simulink model "VisualizationData"  (R2020a)
settings: Solver=VariableStepAuto  StartTime=0.0  StopTime=60  RelTol=1e-3
settings Model: Creator=kashy  LastModifiedBy=kashy

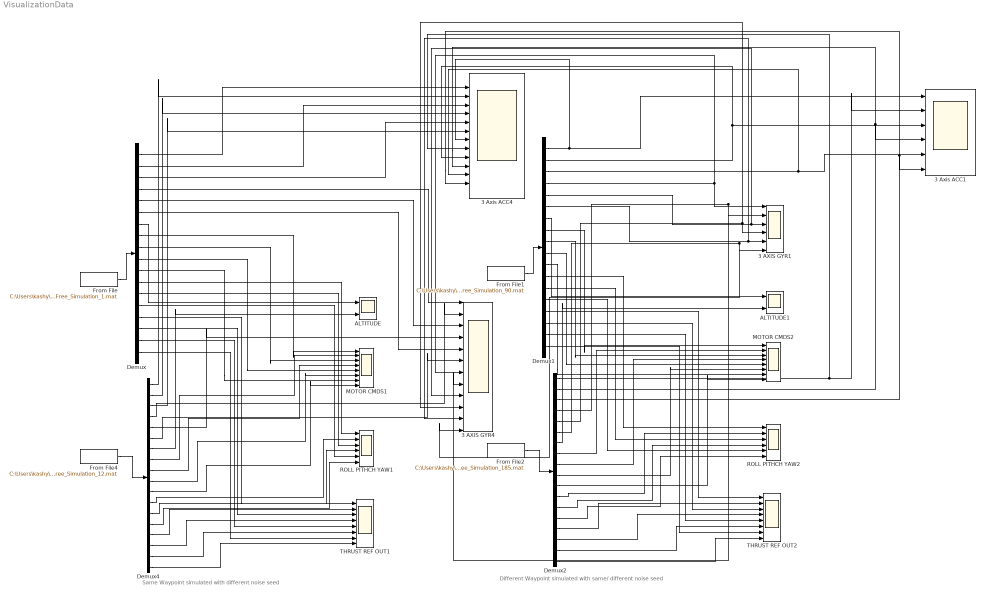
== system VisualizationData ==
  note: Same Waypoint simulated with different noise seed
  note: Different Waypoint simulated with same/ different noise seed
  3 AXIS GYR1 : Scope  NumInputPorts=6
  3 AXIS GYR4 : Scope  NumInputPorts=12
  3 Axis ACC1 : Scope  NumInputPorts=6
  3 Axis ACC4 : Scope  NumInputPorts=12
  ALTITUDE : Scope  NumInputPorts=2
  ALTITUDE1 : Scope  NumInputPorts=2
  Demux{,1..2,4} (4 alike) : Demux  Outputs=18
  From File : FromFile  FileName=C:\Users\kashy\Documents\MATLAB\Master_Thesis\model\parrotMinidroneWaypointFollower\Fault_Free_Data\Fault_Free_Simulation_1.mat  SampleTime=0.1
  From File1 : FromFile  FileName=C:\Users\kashy\Documents\MATLAB\Master_Thesis\model\parrotMinidroneWaypointFollower\Fault_Free_Data\Fault_Free_Simulation_90.mat  SampleTime=0.1
  From File2 : FromFile  FileName=C:\Users\kashy\Documents\MATLAB\Master_Thesis\model\parrotMinidroneWaypointFollower\Fault_Free_Data\Fault_Free_Simulation_185.mat  SampleTime=0.1
  From File4 : FromFile  FileName=C:\Users\kashy\Documents\MATLAB\Master_Thesis\model\parrotMinidroneWaypointFollower\Fault_Free_Data\Fault_Free_Simulation_12.mat  SampleTime=0.1
  MOTOR CMDS1 : Scope  NumInputPorts=8
  MOTOR CMDS2 : Scope  NumInputPorts=8
  ROLL PITHCH YAW1 : Scope  NumInputPorts=6
  ROLL PITHCH YAW2 : Scope  NumInputPorts=6
  THRUST REF OUT1 : Scope  NumInputPorts=8
  THRUST REF OUT2 : Scope  NumInputPorts=8
  wires:
  From File/1 -> Demux/1
  Demux/7 -> ALTITUDE/1
  From File4/1 -> Demux4/1
  Demux/1 -> 3 Axis ACC4/1
  Demux4/1 -> 3 Axis ACC4/2
  Demux/2 -> 3 Axis ACC4/3
  Demux4/2 -> 3 Axis ACC4/4
  Demux/3 -> 3 Axis ACC4/5
  Demux4/3 -> 3 Axis ACC4/6
  Demux/4 -> 3 AXIS GYR4/1
  Demux4/4 -> 3 AXIS GYR4/2
  Demux/5 -> 3 AXIS GYR4/3
  Demux4/5 -> 3 AXIS GYR4/4
  Demux/6 -> 3 AXIS GYR4/5
  Demux4/6 -> 3 AXIS GYR4/6
  Demux4/7 -> ALTITUDE/2
  Demux/8 -> MOTOR CMDS1/1
  Demux4/8 -> MOTOR CMDS1/2
  Demux/9 -> MOTOR CMDS1/3
  Demux4/9 -> MOTOR CMDS1/4
  Demux/10 -> MOTOR CMDS1/5
  Demux4/10 -> MOTOR CMDS1/6
  Demux/11 -> MOTOR CMDS1/7
  Demux4/11 -> MOTOR CMDS1/8
  Demux/12 -> ROLL PITHCH YAW1/1
  Demux4/12 -> ROLL PITHCH YAW1/2
  Demux/13 -> ROLL PITHCH YAW1/3
  Demux4/13 -> ROLL PITHCH YAW1/4
  Demux/14 -> ROLL PITHCH YAW1/5
  Demux4/14 -> ROLL PITHCH YAW1/6
  Demux/15 -> THRUST REF OUT1/1
  Demux4/15 -> THRUST REF OUT1/2
  Demux/16 -> THRUST REF OUT1/3
  Demux4/16 -> THRUST REF OUT1/4
  Demux/17 -> THRUST REF OUT1/5
  Demux4/17 -> THRUST REF OUT1/6
  Demux/18 -> THRUST REF OUT1/7
  Demux4/18 -> THRUST REF OUT1/8
  Demux1/10 -> MOTOR CMDS2/5
  Demux1/15 -> THRUST REF OUT2/1
  Demux1/18 -> THRUST REF OUT2/7
  Demux2/8 -> MOTOR CMDS2/2
  From File2/1 -> Demux2/1
  Demux1/1 -> 3 Axis ACC4/7, 3 Axis ACC1/1
  Demux2/18 -> THRUST REF OUT2/8
  Demux2/9 -> MOTOR CMDS2/4
  Demux1/9 -> MOTOR CMDS2/3
  Demux2/17 -> THRUST REF OUT2/6
  Demux2/13 -> ROLL PITHCH YAW2/4
  Demux2/14 -> ROLL PITHCH YAW2/6
  Demux1/3 -> 3 Axis ACC4/11, 3 Axis ACC1/5
  Demux2/11 -> MOTOR CMDS2/8
  Demux2/10 -> MOTOR CMDS2/6
  Demux1/8 -> MOTOR CMDS2/1
  Demux2/6 -> 3 AXIS GYR4/12, 3 AXIS GYR1/6
  Demux2/5 -> 3 AXIS GYR4/10, 3 AXIS GYR1/4
  Demux2/12 -> ROLL PITHCH YAW2/2
  Demux2/2 -> 3 Axis ACC4/10, 3 Axis ACC1/4
  Demux1/5 -> 3 AXIS GYR4/9, 3 AXIS GYR1/3
  Demux1/17 -> THRUST REF OUT2/5
  Demux2/4 -> 3 AXIS GYR4/8, 3 AXIS GYR1/2
  Demux1/16 -> THRUST REF OUT2/3
  Demux1/12 -> ROLL PITHCH YAW2/1
  Demux1/6 -> 3 AXIS GYR4/11, 3 AXIS GYR1/5
  Demux1/7 -> ALTITUDE1/1
  Demux2/7 -> ALTITUDE1/2
  Demux2/3 -> 3 Axis ACC4/12, 3 Axis ACC1/6
  Demux2/15 -> THRUST REF OUT2/2
  Demux1/2 -> 3 Axis ACC4/9, 3 Axis ACC1/3
  Demux1/4 -> 3 AXIS GYR1/1, 3 AXIS GYR4/7
  Demux1/14 -> ROLL PITHCH YAW2/5
  Demux2/1 -> 3 Axis ACC4/8, 3 Axis ACC1/2
  Demux1/11 -> MOTOR CMDS2/7
  From File1/1 -> Demux1/1
  Demux1/13 -> ROLL PITHCH YAW2/3
  Demux2/16 -> THRUST REF OUT2/4
